simulink model "friction"  (R2022a)
settings: Solver=VariableStepAuto  StartTime=0.0  StopTime=10.0  RelTol=1e-3
libraries: simulink x1
settings Model: Creator=farfar  LastModifiedBy=farfar
settings DataIOCC: ReturnWorkspaceOutputs=off

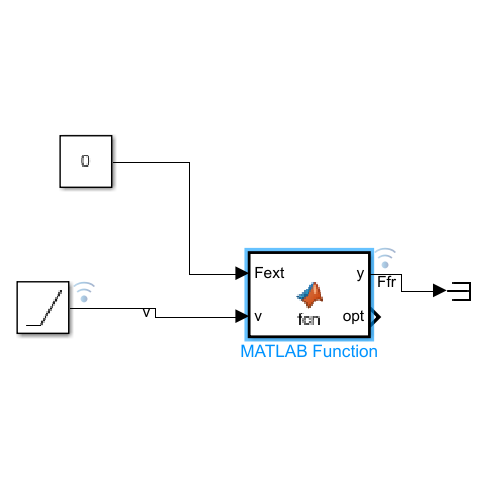
[thumbnail: Simulink's stored preview of the top-level diagram]
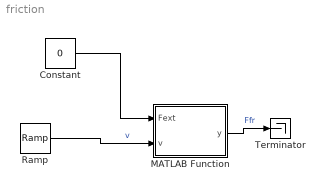
== system friction ==
  Constant : Constant  Value=0
  MATLAB Function : MATLAB Function  TreatAsAtomicUnit=on
  Ramp : simulink/Sources/Ramp  slope=1  start=0  InitialOutput=-10
  Terminator : Terminator
  wires:
  Ramp/1 -> MATLAB Function/2(v)  "v"
  Constant/1 -> MATLAB Function/1(Fext)
  MATLAB Function/1(y) -> Terminator/1  "Ffr"

== matlab function friction/MATLAB Function ==
  data: Fext input; y output; v input
function y = fcn(Fext, v)
mu_s = 1;
mu_k = 0.5;
mu_v = 0.3;
a_st = 1;
FN = 3;
Fs = mu_s * FN;% * sign(v);
Fk = mu_k * FN;% * sign(v);
Fv = 0;%mu_v * FN;

v_tol = 0.0001;
y = 0;
opt = 0;
if and(abs(v) <= v_tol, Fext < Fs)
    y = Fext;
    opt = 1;
elseif and(abs(v) <= v_tol, Fext >= Fs)
    y = Fs;
    opt = 2;
elseif and(abs(v) > v_tol, v > 0)
    y = Fk + (Fs - Fk)*exp(-a_st * v) + Fv * v;
    opt = 3;
elseif and(abs(v) > v_tol, v < 0) 
    y = -Fk + (Fk - Fs)*exp(a_st * v) - Fv * v;
    opt = 4;
end
